simulink model "nonlin"  (R2023a)
settings: Solver=VariableStepAuto  StartTime=0.0  StopTime=10.0  RelTol=1e-3
values from neighbouring files (symbols this model uses):
  g = 9.81    [Initialisation.m]
  J_m = 3.9001*10^(-07)    (= 3.9001e-07)    [Initialisation.m]
  K_g = 70    [Initialisation.m]
  k_t = 0.0076830    (= 0.007683)    [Initialisation.m]
  L = 0.4254    [Initialisation.m]
  m_s = 0.0640    (= 0.064)    [Initialisation.m]
  n_g = 0.9000    (= 0.9)    [Initialisation.m]
  n_m = 0.69    [Initialisation.m]
  r_arm = 0.0254    [Initialisation.m]
  R_m = Iden.R_m    [Initialisation.m]
undefined symbols (not defined in the file or in its folder): B_m, L_m
settings Model: Creator=Mathys  LastModifiedBy=Mathys

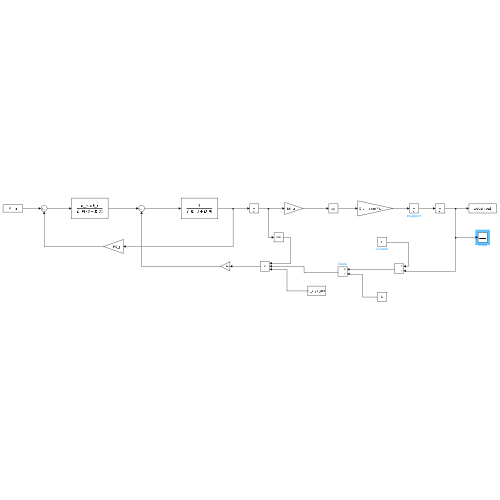
[thumbnail: Simulink's stored preview of the top-level diagram]
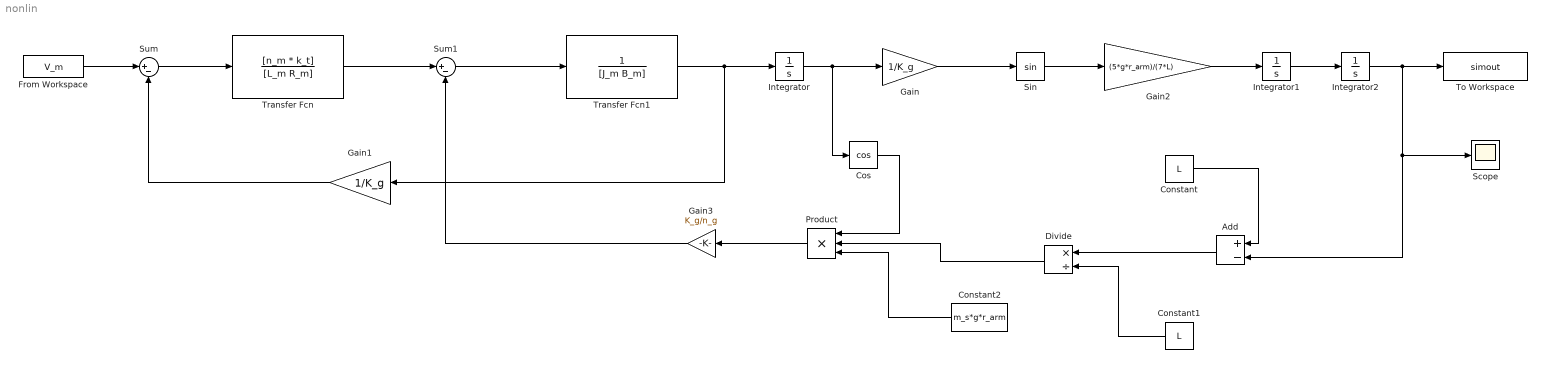
== system nonlin ==
  Add : Sum  Inputs=+-
  Constant : Constant  Value=L
  Constant1 : Constant  Value=L
  Constant2 : Constant  Value=m_s*g*r_arm
  Cos : Trigonometry  Operator=cos
  Divide : Product  Inputs=*/
  From Workspace : FromWorkspace  VariableName=V_m
  Gain : Gain  Gain=1/K_g
  Gain1 : Gain  Gain=1/K_g
  Gain2 : Gain  Gain=(5*g*r_arm)/(7*L)
  Gain3 : Gain  Gain=K_g/n_g
  Integrator : Integrator
  Integrator1 : Integrator
  Integrator2 : Integrator
  Product : Product  Inputs=3
  Scope : Scope
  Sin : Trigonometry
  Sum : Sum  Inputs=|+-
  Sum1 : Sum  Inputs=|+-
  To Workspace : ToWorkspace  VariableName=simout  SaveFormat=Timeseries  SampleTime=-1
  Transfer Fcn : TransferFcn  Numerator=[n_m * k_t]  Denominator=[L_m R_m]
  Transfer Fcn1 : TransferFcn  Denominator=[J_m B_m]
  wires:
  From Workspace/1 -> Sum/1
  Sum/1 -> Transfer Fcn/1
  Transfer Fcn/1 -> Sum1/1
  Sum1/1 -> Transfer Fcn1/1
  Transfer Fcn1/1 -> Gain1/1, Integrator/1
  Integrator/1 -> Cos/1, Gain/1
  Gain1/1 -> Sum/2
  Gain/1 -> Sin/1
  Sin/1 -> Gain2/1
  Gain2/1 -> Integrator1/1
  Integrator1/1 -> Integrator2/1
  Integrator2/1 -> Add/2, Scope/1, To Workspace/1
  Gain3/1 -> Sum1/2
  Constant/1 -> Add/1
  Add/1 -> Divide/1
  Constant1/1 -> Divide/2
  Cos/1 -> Product/1
  Divide/1 -> Product/2
  Constant2/1 -> Product/3
  Product/1 -> Gain3/1
